simulink model "velo_pi_mbd_simu"  (R2020b)
settings: Solver=VariableStepAuto  StartTime=0.0  StopTime=t_end  RelTol=1e-3
values from neighbouring files (symbols this model uses):
  K = K_id    [velo_pi_mbd.m]
  Ki = p1*p2*T/K    [velo_pi_mbd.m]
  Kp = -((p1+p2)*T + 1)/K    [velo_pi_mbd.m]
  T = T_id    [velo_pi_mbd.m]
libraries: arduino_io_lib x4
settings Model: Creator=kei55  LastModifiedBy=kei55

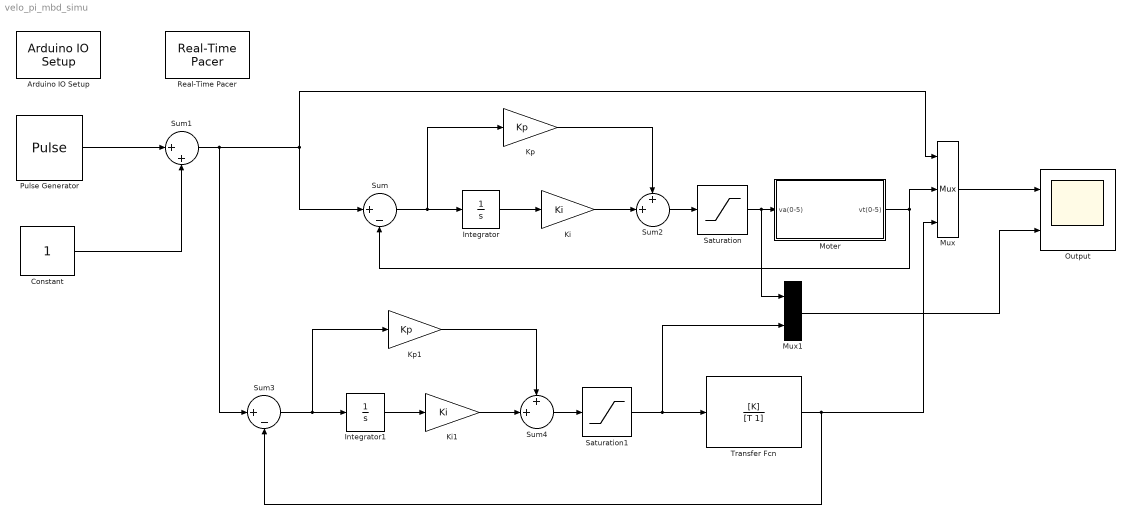
== system velo_pi_mbd_simu ==
  Arduino IO Setup : arduino_io_lib/Arduino IO Setup  Priority=3  arduinoVar=Temporary arduino variable: Arduino1  workspaceVarName=a  comPort=COM3
  Constant : Constant
  Integrator : Integrator
  Integrator1 : Integrator
  Ki : Gain  Gain=Ki
  Ki1 : Gain  Gain=Ki
  Kp : Gain  Gain=Kp
  Kp1 : Gain  Gain=Kp
  Moter : Subsystem
  Mux : Mux  Inputs=3
  Mux1 : Mux  Inputs=2
  Output : Scope  NumInputPorts=2
  Pulse Generator : DiscretePulseGenerator  PulseType=Time based  Amplitude=0.5  Period=4  PulseWidth=50  SampleTime=1/50
  Real-Time Pacer : arduino_io_lib/Real-Time Pacer  simTimePerRealTime=1
  Saturation : Saturate  UpperLimit=5  LowerLimit=0
  Saturation1 : Saturate  UpperLimit=5  LowerLimit=0
  Sum : Sum  Inputs=|+-
  Sum1 : Sum  Inputs=|++
  Sum2 : Sum  Inputs=++|
  Sum3 : Sum  Inputs=|+-
  Sum4 : Sum  Inputs=++|
  Transfer Fcn : TransferFcn  Numerator=[K]  Denominator=[T 1]
  wires:
  Mux/1 -> Output/1
  Moter/1(vt(0-5)) -> Sum/2, Mux/2
  Pulse Generator/1 -> Sum1/1
  Constant/1 -> Sum1/2
  Integrator/1 -> Ki/1
  Sum1/1 -> Sum/1, Mux/1, Sum3/1
  Sum/1 -> Kp/1, Integrator/1
  Kp/1 -> Sum2/1
  Ki/1 -> Sum2/2
  Sum2/1 -> Saturation/1
  Saturation/1 -> Mux1/1, Moter/1(va(0-5))
  Kp1/1 -> Sum4/1
  Ki1/1 -> Sum4/2
  Saturation1/1 -> Mux1/2, Transfer Fcn/1
  Sum4/1 -> Saturation1/1
  Sum3/1 -> Kp1/1, Integrator1/1
  Integrator1/1 -> Ki1/1
  Transfer Fcn/1 -> Mux/3, Sum3/2
  Mux1/1 -> Output/2

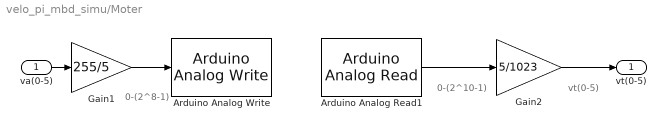
== system velo_pi_mbd_simu/Moter ==
  note: 0-(2^8-1)
  note: 0-(2^10-1)
  note: vt(0-5)
  va(0-5) : Inport
  Arduino Analog Read1 : arduino_io_lib/Arduino Analog Read  arduinoVar=Temporary arduino variable: Arduino1  arduinoPin=0  T=1/50
  Arduino Analog Write : arduino_io_lib/Arduino Analog Write  arduinoVar=Temporary arduino variable: Arduino1  arduinoPin=3  T=1/50
  Gain1 : Gain  Gain=255/5
  Gain2 : Gain  Gain=5/1023
  vt(0-5) : Outport
  wires:
  Arduino Analog Read1/1 -> Gain2/1
  Gain1/1 -> Arduino Analog Write/1
  Gain2/1 -> vt(0-5)/1
  va(0-5)/1 -> Gain1/1
